simulink model "cal_2adc"  (R2012b)
settings: Solver=ode45  StartTime=0.0  StopTime=10.0  RelTol=1e-3
libraries: xbsIndex_r4 x665, dspsigops x32, xps_library x1
(part 1 of 5)
settings Model: Creator=rprimian  LastModifiedBy=root
settings DataIOCC: SignalLoggingSaveFormat=ModelDataLogs
settings DebuggingCC: SolverPrmCheckMsg=none  FcnCallInpInsideContextMsg=UseLocalSettings  StrictBusMsg=Warning
settings GRTTargetCC: CombineOutputUpdateFcns=off  GRTInterface=on

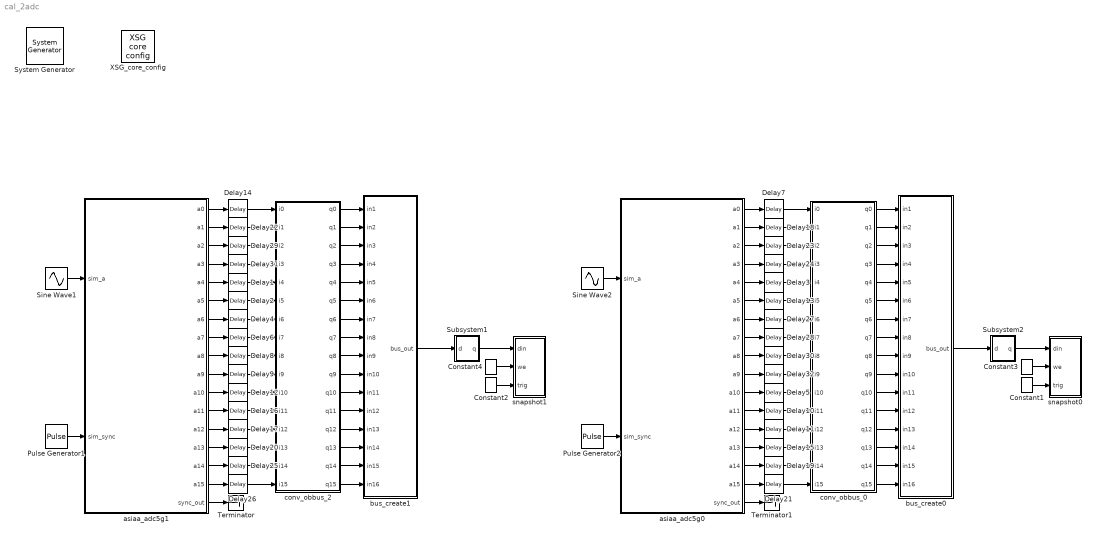
== system cal_2adc ==
  " System Generator" : xbsIndex_r4/ System Generator  Tag=genX  xilinxfamily=virtex6  part=xc6vsx475t  speed=-1  package=ff1759  synthesis_tool=XST  clock_wrapper=Clock Enables  directory=./cal_2adc/sysgen  proj_type=Project Navigator  Synth_file=XST Defaults  Impl_file=ISE Defaults  testbench=off  simulink_period=1  sysclk_period=4  dcm_input_clock_period=100  incr_netlist=off  trim_vbits=Everywhere in SubSystem  dbl_ovrd=According to Block Masks  core_generation=According to Block Masks  run_coregen=off  deprecated_control=off  eval_field=0  block_type=sysgen
  Constant{1..4} (4 alike) : xbsIndex_r4/Constant  const=1  gui_display_data_type=Fixed-point  arith_type=Boolean  n_bits=16  bin_pt=14  preci_type=Single  exp_width=8  frac_width=24  explicit_period=on  period=1  equ=P=C  opselect=C  inp2=PCIN>>17  opr=+  inp1=P  carry=CIN  dbl_ovrd=off  block_type=constant
      settings: block_version=11.4
  Delay{1..32} (32 alike) : xbsIndex_r4/Delay  rst=off  infoeditControl=Selection of Reset will increase slice count due to use of real FFs and instead of SRLs  en=off  latency=2  dbl_ovrd=off  reg_retiming=off  block_type=delay
  Pulse Generator1 : DiscretePulseGenerator  Period=1000
  Pulse Generator2 : DiscretePulseGenerator  Period=1000
  Sine Wave1 : Sin  SineType=Sample based  SampleTime=1/8
  Sine Wave2 : Sin  SineType=Sample based  SampleTime=1/8
  Subsystem1 : Subsystem
  Subsystem2 : Subsystem
  Terminator : Terminator
  Terminator1 : Terminator
  XSG_core_config : xps_library/XSG core config  Tag=xps:xsg  hw_sys=ROACH2:sx475t  clk_src=adc1_clk  ROACH_clk_src=adc0_clk  ROACH2_clk_src=adc1_clk  clk_rate=250  sample_period=1  synthesis_tool=XST
  asiaa_adc5g0 : Subsystem  Tag=xps:adc5g  AncestorBlock=xps_library/ADCs/asiaa_adc5g  mask(adc5g){input_mode=One-channel -- A, adc_brd=ZDOK 0, demux=1:1, adc_bit_width=8, adc_clk_rate=1200, using_ctrl=on, test_ramp=off}
      mask prompts: input_mode "Input mode:"; adc_brd "ADC Board"; demux "Internal demux"; adc_bit_width "ADC Resolution (bits):"; adc_clk_rate "ADC Clock Rate (MHz):"; using_ctrl "use control"; test_ramp "start in test ramp mode"
      mask help:
      | Interface for the ASIAA 5 GSps ADC. Supports interleaving all four
      | cores using either input A or C, or interleaving two-cores each for
      | A and C. The hardware itself comes in two versions:
      |
      | DMUX 1:2 -- 4-bit samples, 4 parallel streams
      | DMUX 1:1 -- 8-bit samples, 2 parallel streams
      |
      | In either configuration this block will output 8 parallel streams
      | but the underlying interface, and the bitwidth of the samples,
      | will be different.
      mask init:
      | adc5g_init(gcb,...
      |     'input_mode', input_mode,...
      |     'demux', demux,...
      |     'adc_clk_rate', adc_clk_rate,...
      |     'adc_bit_width', adc_bit_width,...
      |     'adc_brd', adc_brd,...
      |     'using_ctrl', using_ctrl,...
      |     'test_ramp', test_ramp);
      mask TypeOptions input_mode: One-channel -- A | One-channel -- C | Two-channel -- A&C
      mask TypeOptions adc_brd: ZDOK 0 | ZDOK 1
      mask TypeOptions demux: 1:1 | 1:2
      mask Callback demux:
      | demux = get_param(gcb,'demux');
      | if(strcmp(demux,'1:1')),
      |     set_param(gcb, 'adc_bit_width', '8')
      | elseif(strcmp(demux, '1:2')),
      |     set_param(gcb, 'adc_bit_width', '4');
      | else
      | end
  asiaa_adc5g1 : Subsystem  Tag=xps:adc5g  AncestorBlock=xps_library/ADCs/asiaa_adc5g  mask(adc5g){input_mode=One-channel -- A, adc_brd=ZDOK 1, demux=1:1, adc_bit_width=8, adc_clk_rate=1800, using_ctrl=on, test_ramp=off}
      mask prompts: input_mode "Input mode:"; adc_brd "ADC Board"; demux "Internal demux"; adc_bit_width "ADC Resolution (bits):"; adc_clk_rate "ADC Clock Rate (MHz):"; using_ctrl "use control"; test_ramp "start in test ramp mode"
      mask help:
      | Interface for the ASIAA 5 GSps ADC. Supports interleaving all four
      | cores using either input A or C, or interleaving two-cores each for
      | A and C. The hardware itself comes in two versions:
      |
      | DMUX 1:2 -- 4-bit samples, 4 parallel streams
      | DMUX 1:1 -- 8-bit samples, 2 parallel streams
      |
      | In either configuration this block will output 8 parallel streams
      | but the underlying interface, and the bitwidth of the samples,
      | will be different.
      mask init: same as cal_2adc/asiaa_adc5g0
      mask TypeOptions input_mode: One-channel -- A | One-channel -- C | Two-channel -- A&C
      mask TypeOptions adc_brd: ZDOK 0 | ZDOK 1
      mask TypeOptions demux: 1:1 | 1:2
      mask Callback demux:
      | demux = get_param(gcb,'demux');
      | if(strcmp(demux,'1:1')),
      |     set_param(gcb, 'adc_bit_width', '8')
      | elseif(strcmp(demux, '1:2')),
      |     set_param(gcb, 'adc_bit_width', '4');
      | else
      | end
  bus_create0 : Subsystem  AncestorBlock=casper_library_flow_control/bus_create  mask(bus_create){inputNum=16}
      mask prompts: inputNum "Number of inputs:"
      mask init:
      | bus_create_init(gcb,...
      |     'inputNum', inputNum);
  bus_create1 : Subsystem  AncestorBlock=casper_library_flow_control/bus_create  mask(bus_create){inputNum=16}
      mask prompts: inputNum "Number of inputs:"
      mask init:
      | bus_create_init(gcb,...
      |     'inputNum', inputNum);
  conv_obbus_0 : Subsystem
  conv_obbus_2 : Subsystem
  snapshot0 : Subsystem  Tag=casper:snapshot  AncestorBlock=casper_library_scopes/snapshot  mask(snapshot){storage=bram, dram_dimm=1, dram_clock=200, nsamples=10, data_width=128, offset=on, circap=off, value=off, use_dsp48=on}
      mask prompts: storage "Storage medium"; dram_dimm "DRAM dimm"; dram_clock "DRAM clock rate"; nsamples "Number of Samples (2^?)"; data_width "Data width"; offset "Start delay support"; circap "Circular capture support"; value "Extra value capture support"; use_dsp48 "Use DSP48s to implement counters"
      mask help:
      | Standard snap block, but with the following optional extras;
      |  1) Optionally delay the fabric trigger by a user-specified number of valids.
      |  2) Capture continuously after a trigger until a stop pulse is received. Data is captured into BRAM continuously, with old data being overwritten until a stop command is received. Then stop capturing when memory is filled. This enables you to get some data before and some data after the stop pulse. Use the 'tr_en_cnt' register to determine where you are in your vector. 'Addr' register's MSb now indicates 'busy capturing'.
      |  3) Optionally capture a value on an input port to a register at the same time as the first data sample.
      |  4) Implement counters using DSP48Es to save resources.
      mask init:
      | snapshot_init(gcb, ...
      |     'storage', storage, ...
      |     'dram_dimm', dram_dimm, ...
      |     'dram_clock', dram_clock, ...
      |     'nsamples', nsamples, ...
      |     'data_width', data_width, ...
      |     'offset', offset, ...
      |     'circap', circap, ...
      |     'value', value, ...
      |     'use_dsp48', use_dsp48);
      mask TypeOptions storage: bram | dram
      mask Callback storage: snapshot_callback();
      mask TypeOptions dram_dimm: 1 | 2 | 3 | 4
      mask TypeOptions dram_clock: 200 | 250 | 266 | 300 | 333
      mask TypeOptions data_width: 8 | 16 | 32 | 64 | 128
  snapshot1 : Subsystem  Tag=casper:snapshot  AncestorBlock=casper_library_scopes/snapshot  mask(snapshot){storage=bram, dram_dimm=1, dram_clock=200, nsamples=10, data_width=128, offset=on, circap=off, value=off, use_dsp48=on}
      mask prompts: storage "Storage medium"; dram_dimm "DRAM dimm"; dram_clock "DRAM clock rate"; nsamples "Number of Samples (2^?)"; data_width "Data width"; offset "Start delay support"; circap "Circular capture support"; value "Extra value capture support"; use_dsp48 "Use DSP48s to implement counters"
      mask help:
      | Standard snap block, but with the following optional extras;
      |  1) Optionally delay the fabric trigger by a user-specified number of valids.
      |  2) Capture continuously after a trigger until a stop pulse is received. Data is captured into BRAM continuously, with old data being overwritten until a stop command is received. Then stop capturing when memory is filled. This enables you to get some data before and some data after the stop pulse. Use the 'tr_en_cnt' register to determine where you are in your vector. 'Addr' register's MSb now indicates 'busy capturing'.
      |  3) Optionally capture a value on an input port to a register at the same time as the first data sample.
      |  4) Implement counters using DSP48Es to save resources.
      mask init: same as cal_2adc/snapshot0
      mask TypeOptions storage: bram | dram
      mask Callback storage: snapshot_callback();
      mask TypeOptions dram_dimm: 1 | 2 | 3 | 4
      mask TypeOptions dram_clock: 200 | 250 | 266 | 300 | 333
      mask TypeOptions data_width: 8 | 16 | 32 | 64 | 128
  wires:
  Constant4/1 -> snapshot1/2(we)
  Pulse Generator1/1 -> asiaa_adc5g1/2(sim_sync)
  Sine Wave1/1 -> asiaa_adc5g1/1(sim_a)
  Subsystem1/1(q) -> snapshot1/1(din)
  Constant2/1 -> snapshot1/3(trig)
  asiaa_adc5g1/17(sync_out) -> Terminator/1
  asiaa_adc5g1/11(a10) -> Delay12/1
  asiaa_adc5g1/12(a11) -> Delay16/1
  asiaa_adc5g1/13(a12) -> Delay17/1
  asiaa_adc5g1/14(a13) -> Delay20/1
  asiaa_adc5g1/1(a0) -> Delay14/1
  asiaa_adc5g1/2(a1) -> Delay22/1
  asiaa_adc5g1/3(a2) -> Delay29/1
  asiaa_adc5g1/4(a3) -> Delay31/1
  asiaa_adc5g1/5(a4) -> Delay1/1
  asiaa_adc5g1/6(a5) -> Delay2/1
  asiaa_adc5g1/7(a6) -> Delay4/1
  asiaa_adc5g1/8(a7) -> Delay6/1
  asiaa_adc5g1/9(a8) -> Delay8/1
  asiaa_adc5g1/10(a9) -> Delay9/1
  asiaa_adc5g1/15(a14) -> Delay25/1
  asiaa_adc5g1/16(a15) -> Delay26/1
  bus_create1/1(bus_out) -> Subsystem1/1(d)
  Delay29/1 -> conv_obbus_2/3(i2)
  Delay8/1 -> conv_obbus_2/9(i8)
  Delay4/1 -> conv_obbus_2/7(i6)
  Delay9/1 -> conv_obbus_2/10(i9)
  Delay6/1 -> conv_obbus_2/8(i7)
  Delay16/1 -> conv_obbus_2/12(i11)
  Delay12/1 -> conv_obbus_2/11(i10)
  Delay17/1 -> conv_obbus_2/13(i12)
  Delay2/1 -> conv_obbus_2/6(i5)
  Delay22/1 -> conv_obbus_2/2(i1)
  Delay20/1 -> conv_obbus_2/14(i13)
  Delay31/1 -> conv_obbus_2/4(i3)
  Delay14/1 -> conv_obbus_2/1(i0)
  Delay25/1 -> conv_obbus_2/15(i14)
  Delay26/1 -> conv_obbus_2/16(i15)
  Delay1/1 -> conv_obbus_2/5(i4)
  conv_obbus_2/5(q4) -> bus_create1/5(in5)
  conv_obbus_2/7(q6) -> bus_create1/7(in7)
  conv_obbus_2/2(q1) -> bus_create1/2(in2)
  conv_obbus_2/11(q10) -> bus_create1/11(in11)
  conv_obbus_2/8(q7) -> bus_create1/8(in8)
  conv_obbus_2/13(q12) -> bus_create1/13(in13)
  conv_obbus_2/4(q3) -> bus_create1/4(in4)
  conv_obbus_2/15(q14) -> bus_create1/15(in15)
  conv_obbus_2/16(q15) -> bus_create1/16(in16)
  conv_obbus_2/12(q11) -> bus_create1/12(in12)
  conv_obbus_2/6(q5) -> bus_create1/6(in6)
  conv_obbus_2/14(q13) -> bus_create1/14(in14)
  conv_obbus_2/1(q0) -> bus_create1/1(in1)
  conv_obbus_2/10(q9) -> bus_create1/10(in10)
  conv_obbus_2/9(q8) -> bus_create1/9(in9)
  conv_obbus_2/3(q2) -> bus_create1/3(in3)
  Constant3/1 -> snapshot0/2(we)
  Pulse Generator2/1 -> asiaa_adc5g0/2(sim_sync)
  Sine Wave2/1 -> asiaa_adc5g0/1(sim_a)
  Subsystem2/1(q) -> snapshot0/1(din)
  Constant1/1 -> snapshot0/3(trig)
  asiaa_adc5g0/17(sync_out) -> Terminator1/1
  asiaa_adc5g0/11(a10) -> Delay5/1
  asiaa_adc5g0/12(a11) -> Delay10/1
  asiaa_adc5g0/13(a12) -> Delay11/1
  asiaa_adc5g0/14(a13) -> Delay15/1
  asiaa_adc5g0/1(a0) -> Delay7/1
  asiaa_adc5g0/2(a1) -> Delay18/1
  asiaa_adc5g0/3(a2) -> Delay23/1
  asiaa_adc5g0/4(a3) -> Delay24/1
  asiaa_adc5g0/5(a4) -> Delay3/1
  asiaa_adc5g0/6(a5) -> Delay13/1
  asiaa_adc5g0/7(a6) -> Delay27/1
  asiaa_adc5g0/8(a7) -> Delay28/1
  asiaa_adc5g0/9(a8) -> Delay30/1
  asiaa_adc5g0/10(a9) -> Delay32/1
  asiaa_adc5g0/15(a14) -> Delay19/1
  asiaa_adc5g0/16(a15) -> Delay21/1
  bus_create0/1(bus_out) -> Subsystem2/1(d)
  Delay23/1 -> conv_obbus_0/3(i2)
  Delay30/1 -> conv_obbus_0/9(i8)
  Delay27/1 -> conv_obbus_0/7(i6)
  Delay32/1 -> conv_obbus_0/10(i9)
  Delay28/1 -> conv_obbus_0/8(i7)
  Delay10/1 -> conv_obbus_0/12(i11)
  Delay5/1 -> conv_obbus_0/11(i10)
  Delay11/1 -> conv_obbus_0/13(i12)
  Delay13/1 -> conv_obbus_0/6(i5)
  Delay18/1 -> conv_obbus_0/2(i1)
  Delay15/1 -> conv_obbus_0/14(i13)
  Delay24/1 -> conv_obbus_0/4(i3)
  Delay7/1 -> conv_obbus_0/1(i0)
  Delay19/1 -> conv_obbus_0/15(i14)
  Delay21/1 -> conv_obbus_0/16(i15)
  Delay3/1 -> conv_obbus_0/5(i4)
  conv_obbus_0/5(q4) -> bus_create0/5(in5)
  conv_obbus_0/7(q6) -> bus_create0/7(in7)
  conv_obbus_0/2(q1) -> bus_create0/2(in2)
  conv_obbus_0/11(q10) -> bus_create0/11(in11)
  conv_obbus_0/8(q7) -> bus_create0/8(in8)
  conv_obbus_0/13(q12) -> bus_create0/13(in13)
  conv_obbus_0/4(q3) -> bus_create0/4(in4)
  conv_obbus_0/15(q14) -> bus_create0/15(in15)
  conv_obbus_0/16(q15) -> bus_create0/16(in16)
  conv_obbus_0/12(q11) -> bus_create0/12(in12)
  conv_obbus_0/6(q5) -> bus_create0/6(in6)
  conv_obbus_0/14(q13) -> bus_create0/14(in14)
  conv_obbus_0/1(q0) -> bus_create0/1(in1)
  conv_obbus_0/10(q9) -> bus_create0/10(in10)
  conv_obbus_0/9(q8) -> bus_create0/9(in9)
  conv_obbus_0/3(q2) -> bus_create0/3(in3)

== system cal_2adc/Subsystem1 ==
  d : Inport
  Register : xbsIndex_r4/Register  init=0  rst=off  en=off  dbl_ovrd=off  block_type=register
      settings: block_version=11.4
  Register1 : xbsIndex_r4/Register  init=0  rst=off  en=off  dbl_ovrd=off  block_type=register
      settings: block_version=11.4
  q : Outport
  wires:
  Register1/1 -> q/1
  Register/1 -> Register1/1
  d/1 -> Register/1

== system cal_2adc/Subsystem2 ==
  d : Inport
  Register : xbsIndex_r4/Register  init=0  rst=off  en=off  dbl_ovrd=off  block_type=register
      settings: block_version=11.4
  Register1 : xbsIndex_r4/Register  init=0  rst=off  en=off  dbl_ovrd=off  block_type=register
      settings: block_version=11.4
  q : Outport
  wires:
  d/1 -> Register/1
  Register/1 -> Register1/1
  Register1/1 -> q/1

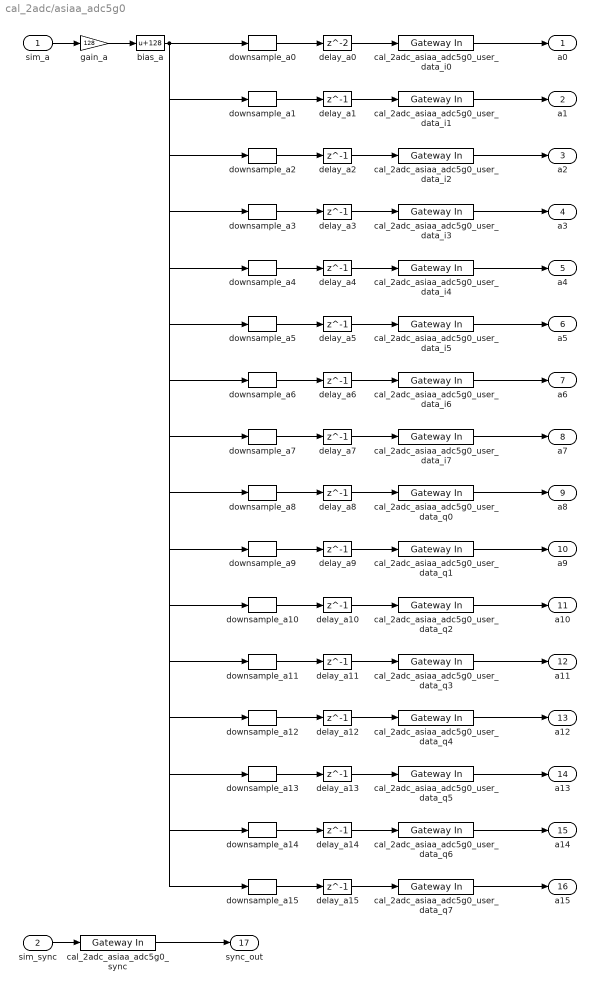
== system cal_2adc/asiaa_adc5g0 ==
  sim_a : Inport
  sim_sync : Inport  Port=2
  bias_a : Bias  Bias=128  SaturateOnIntegerOverflow=on
  cal_2adc_asiaa_adc5g0_sync : xbsIndex_r4/Gateway In  gui_display_data_type=Fixed-point  arith_type=Boolean  n_bits=16  bin_pt=14  preci_type=Single  exp_width=8  frac_width=24  quantization="Round  (unbiased: +/- Inf)"  overflow=Saturate  period=1  dbl_ovrd=off  timing_constraint=None  locs_specified=off  LOCs={}  UseAsADC=off  ADCChannel='1'  inherit_from_input=off  hdl_port=on  block_type=gatewayin
  cal_2adc_asiaa_adc5g0_user_data_i{0..7} (8 alike) : xbsIndex_r4/Gateway In  gui_display_data_type=Fixed-point  arith_type=Unsigned  n_bits=8  bin_pt=0  preci_type=Single  exp_width=8  frac_width=24  quantization=Truncate  overflow=Wrap  period=1  dbl_ovrd=off  timing_constraint=None  locs_specified=off  LOCs={}  UseAsADC=off  ADCChannel='1'  inherit_from_input=off  hdl_port=on  block_type=gatewayin
  cal_2adc_asiaa_adc5g0_user_data_q{0..7} (8 alike) : xbsIndex_r4/Gateway In  gui_display_data_type=Fixed-point  arith_type=Unsigned  n_bits=8  bin_pt=0  preci_type=Single  exp_width=8  frac_width=24  quantization=Truncate  overflow=Wrap  period=1  dbl_ovrd=off  timing_constraint=None  locs_specified=off  LOCs={}  UseAsADC=off  ADCChannel='1'  inherit_from_input=off  hdl_port=on  block_type=gatewayin
  delay_a0 : Delay  InitialCondition=0  InputProcessing=Inherited
  delay_a{1..15} (15 alike) : Delay  DelayLength=1  InitialCondition=0  InputProcessing=Inherited
  downsample_a0 : dspsigops/Downsample  N=16  phase=0  RateOptions=Allow multirate processing  smode=Allow multirate  fmode=Maintain input frame size  ic=0
  downsample_a1 : dspsigops/Downsample  N=16  phase=1  RateOptions=Allow multirate processing  smode=Allow multirate  fmode=Maintain input frame size  ic=0
  downsample_a10 : dspsigops/Downsample  N=16  phase=10  RateOptions=Allow multirate processing  smode=Allow multirate  fmode=Maintain input frame size  ic=0
  downsample_a11 : dspsigops/Downsample  N=16  phase=11  RateOptions=Allow multirate processing  smode=Allow multirate  fmode=Maintain input frame size  ic=0
  downsample_a12 : dspsigops/Downsample  N=16  phase=12  RateOptions=Allow multirate processing  smode=Allow multirate  fmode=Maintain input frame size  ic=0
  downsample_a13 : dspsigops/Downsample  N=16  phase=13  RateOptions=Allow multirate processing  smode=Allow multirate  fmode=Maintain input frame size  ic=0
  downsample_a14 : dspsigops/Downsample  N=16  phase=14  RateOptions=Allow multirate processing  smode=Allow multirate  fmode=Maintain input frame size  ic=0
  downsample_a15 : dspsigops/Downsample  N=16  phase=15  RateOptions=Allow multirate processing  smode=Allow multirate  fmode=Maintain input frame size  ic=0
  downsample_a2 : dspsigops/Downsample  N=16  phase=2  RateOptions=Allow multirate processing  smode=Allow multirate  fmode=Maintain input frame size  ic=0
  downsample_a3 : dspsigops/Downsample  N=16  phase=3  RateOptions=Allow multirate processing  smode=Allow multirate  fmode=Maintain input frame size  ic=0
  downsample_a4 : dspsigops/Downsample  N=16  phase=4  RateOptions=Allow multirate processing  smode=Allow multirate  fmode=Maintain input frame size  ic=0
  downsample_a5 : dspsigops/Downsample  N=16  phase=5  RateOptions=Allow multirate processing  smode=Allow multirate  fmode=Maintain input frame size  ic=0
  downsample_a6 : dspsigops/Downsample  N=16  phase=6  RateOptions=Allow multirate processing  smode=Allow multirate  fmode=Maintain input frame size  ic=0
  downsample_a7 : dspsigops/Downsample  N=16  phase=7  RateOptions=Allow multirate processing  smode=Allow multirate  fmode=Maintain input frame size  ic=0
  downsample_a8 : dspsigops/Downsample  N=16  phase=8  RateOptions=Allow multirate processing  smode=Allow multirate  fmode=Maintain input frame size  ic=0
  downsample_a9 : dspsigops/Downsample  N=16  phase=9  RateOptions=Allow multirate processing  smode=Allow multirate  fmode=Maintain input frame size  ic=0
  gain_a : Gain  Gain=128  SaturateOnIntegerOverflow=on  OutDataTypeStr=Inherit: Same as input  ParamDataTypeStr=Inherit: Same as input
  a0 : Outport
  a1 : Outport  Port=2
  a2 : Outport  Port=3
  a3 : Outport  Port=4
  a4 : Outport  Port=5
  a5 : Outport  Port=6
  a6 : Outport  Port=7
  a7 : Outport  Port=8
  a8 : Outport  Port=9
  a9 : Outport  Port=10
  a10 : Outport  Port=11
  a11 : Outport  Port=12
  a12 : Outport  Port=13
  a13 : Outport  Port=14
  a14 : Outport  Port=15
  a15 : Outport  Port=16
  sync_out : Outport  Port=17
  wires:
  sim_a/1 -> gain_a/1
  gain_a/1 -> bias_a/1
  bias_a/1 -> downsample_a0/1, downsample_a1/1, downsample_a2/1, downsample_a3/1, downsample_a4/1, downsample_a5/1, downsample_a6/1, downsample_a7/1, downsample_a8/1, downsample_a9/1, downsample_a10/1, downsample_a11/1, downsample_a12/1, downsample_a13/1, downsample_a14/1, downsample_a15/1
  downsample_a0/1 -> delay_a0/1
  delay_a0/1 -> cal_2adc_asiaa_adc5g0_user_data_i0/1
  cal_2adc_asiaa_adc5g0_user_data_i0/1 -> a0/1
  downsample_a1/1 -> delay_a1/1
  delay_a1/1 -> cal_2adc_asiaa_adc5g0_user_data_i1/1
  cal_2adc_asiaa_adc5g0_user_data_i1/1 -> a1/1
  downsample_a2/1 -> delay_a2/1
  delay_a2/1 -> cal_2adc_asiaa_adc5g0_user_data_i2/1
  cal_2adc_asiaa_adc5g0_user_data_i2/1 -> a2/1
  downsample_a3/1 -> delay_a3/1
  delay_a3/1 -> cal_2adc_asiaa_adc5g0_user_data_i3/1
  cal_2adc_asiaa_adc5g0_user_data_i3/1 -> a3/1
  downsample_a4/1 -> delay_a4/1
  delay_a4/1 -> cal_2adc_asiaa_adc5g0_user_data_i4/1
  cal_2adc_asiaa_adc5g0_user_data_i4/1 -> a4/1
  downsample_a5/1 -> delay_a5/1
  delay_a5/1 -> cal_2adc_asiaa_adc5g0_user_data_i5/1
  cal_2adc_asiaa_adc5g0_user_data_i5/1 -> a5/1
  downsample_a6/1 -> delay_a6/1
  delay_a6/1 -> cal_2adc_asiaa_adc5g0_user_data_i6/1
  cal_2adc_asiaa_adc5g0_user_data_i6/1 -> a6/1
  downsample_a7/1 -> delay_a7/1
  delay_a7/1 -> cal_2adc_asiaa_adc5g0_user_data_i7/1
  cal_2adc_asiaa_adc5g0_user_data_i7/1 -> a7/1
  downsample_a8/1 -> delay_a8/1
  delay_a8/1 -> cal_2adc_asiaa_adc5g0_user_data_q0/1
  cal_2adc_asiaa_adc5g0_user_data_q0/1 -> a8/1
  downsample_a9/1 -> delay_a9/1
  delay_a9/1 -> cal_2adc_asiaa_adc5g0_user_data_q1/1
  cal_2adc_asiaa_adc5g0_user_data_q1/1 -> a9/1
  downsample_a10/1 -> delay_a10/1
  delay_a10/1 -> cal_2adc_asiaa_adc5g0_user_data_q2/1
  cal_2adc_asiaa_adc5g0_user_data_q2/1 -> a10/1
  downsample_a11/1 -> delay_a11/1
  delay_a11/1 -> cal_2adc_asiaa_adc5g0_user_data_q3/1
  cal_2adc_asiaa_adc5g0_user_data_q3/1 -> a11/1
  downsample_a12/1 -> delay_a12/1
  delay_a12/1 -> cal_2adc_asiaa_adc5g0_user_data_q4/1
  cal_2adc_asiaa_adc5g0_user_data_q4/1 -> a12/1
  downsample_a13/1 -> delay_a13/1
  delay_a13/1 -> cal_2adc_asiaa_adc5g0_user_data_q5/1
  cal_2adc_asiaa_adc5g0_user_data_q5/1 -> a13/1
  downsample_a14/1 -> delay_a14/1
  delay_a14/1 -> cal_2adc_asiaa_adc5g0_user_data_q6/1
  cal_2adc_asiaa_adc5g0_user_data_q6/1 -> a14/1
  downsample_a15/1 -> delay_a15/1
  delay_a15/1 -> cal_2adc_asiaa_adc5g0_user_data_q7/1
  cal_2adc_asiaa_adc5g0_user_data_q7/1 -> a15/1
  sim_sync/1 -> cal_2adc_asiaa_adc5g0_sync/1
  cal_2adc_asiaa_adc5g0_sync/1 -> sync_out/1

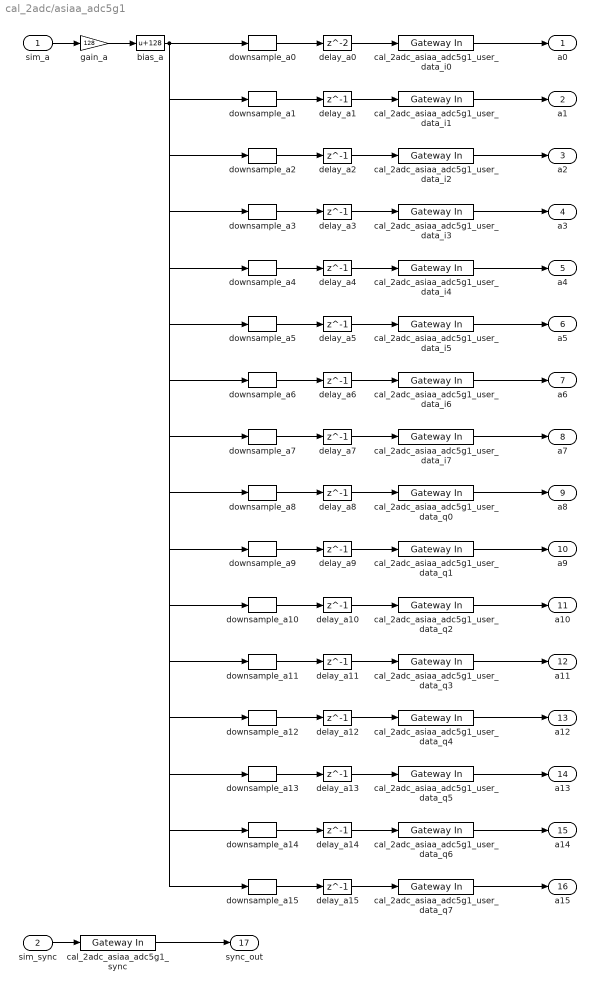
== system cal_2adc/asiaa_adc5g1 ==
  sim_a : Inport
  sim_sync : Inport  Port=2
  bias_a : Bias  Bias=128  SaturateOnIntegerOverflow=on
  cal_2adc_asiaa_adc5g1_sync : xbsIndex_r4/Gateway In  gui_display_data_type=Fixed-point  arith_type=Boolean  n_bits=16  bin_pt=14  preci_type=Single  exp_width=8  frac_width=24  quantization="Round  (unbiased: +/- Inf)"  overflow=Saturate  period=1  dbl_ovrd=off  timing_constraint=None  locs_specified=off  LOCs={}  UseAsADC=off  ADCChannel='1'  inherit_from_input=off  hdl_port=on  block_type=gatewayin
  cal_2adc_asiaa_adc5g1_user_data_i{0..7} (8 alike) : xbsIndex_r4/Gateway In  gui_display_data_type=Fixed-point  arith_type=Unsigned  n_bits=8  bin_pt=0  preci_type=Single  exp_width=8  frac_width=24  quantization=Truncate  overflow=Wrap  period=1  dbl_ovrd=off  timing_constraint=None  locs_specified=off  LOCs={}  UseAsADC=off  ADCChannel='1'  inherit_from_input=off  hdl_port=on  block_type=gatewayin
  cal_2adc_asiaa_adc5g1_user_data_q{0..7} (8 alike) : xbsIndex_r4/Gateway In  gui_display_data_type=Fixed-point  arith_type=Unsigned  n_bits=8  bin_pt=0  preci_type=Single  exp_width=8  frac_width=24  quantization=Truncate  overflow=Wrap  period=1  dbl_ovrd=off  timing_constraint=None  locs_specified=off  LOCs={}  UseAsADC=off  ADCChannel='1'  inherit_from_input=off  hdl_port=on  block_type=gatewayin
  delay_a0 : Delay  InitialCondition=0  InputProcessing=Inherited
  delay_a{1..15} (15 alike) : Delay  DelayLength=1  InitialCondition=0  InputProcessing=Inherited
  downsample_a0 : dspsigops/Downsample  N=16  phase=0  RateOptions=Allow multirate processing  smode=Allow multirate  fmode=Maintain input frame size  ic=0
  downsample_a1 : dspsigops/Downsample  N=16  phase=1  RateOptions=Allow multirate processing  smode=Allow multirate  fmode=Maintain input frame size  ic=0
  downsample_a10 : dspsigops/Downsample  N=16  phase=10  RateOptions=Allow multirate processing  smode=Allow multirate  fmode=Maintain input frame size  ic=0
  downsample_a11 : dspsigops/Downsample  N=16  phase=11  RateOptions=Allow multirate processing  smode=Allow multirate  fmode=Maintain input frame size  ic=0
  downsample_a12 : dspsigops/Downsample  N=16  phase=12  RateOptions=Allow multirate processing  smode=Allow multirate  fmode=Maintain input frame size  ic=0
  downsample_a13 : dspsigops/Downsample  N=16  phase=13  RateOptions=Allow multirate processing  smode=Allow multirate  fmode=Maintain input frame size  ic=0
  downsample_a14 : dspsigops/Downsample  N=16  phase=14  RateOptions=Allow multirate processing  smode=Allow multirate  fmode=Maintain input frame size  ic=0
  downsample_a15 : dspsigops/Downsample  N=16  phase=15  RateOptions=Allow multirate processing  smode=Allow multirate  fmode=Maintain input frame size  ic=0
  downsample_a2 : dspsigops/Downsample  N=16  phase=2  RateOptions=Allow multirate processing  smode=Allow multirate  fmode=Maintain input frame size  ic=0
  downsample_a3 : dspsigops/Downsample  N=16  phase=3  RateOptions=Allow multirate processing  smode=Allow multirate  fmode=Maintain input frame size  ic=0
  downsample_a4 : dspsigops/Downsample  N=16  phase=4  RateOptions=Allow multirate processing  smode=Allow multirate  fmode=Maintain input frame size  ic=0
  downsample_a5 : dspsigops/Downsample  N=16  phase=5  RateOptions=Allow multirate processing  smode=Allow multirate  fmode=Maintain input frame size  ic=0
  downsample_a6 : dspsigops/Downsample  N=16  phase=6  RateOptions=Allow multirate processing  smode=Allow multirate  fmode=Maintain input frame size  ic=0
  downsample_a7 : dspsigops/Downsample  N=16  phase=7  RateOptions=Allow multirate processing  smode=Allow multirate  fmode=Maintain input frame size  ic=0
  downsample_a8 : dspsigops/Downsample  N=16  phase=8  RateOptions=Allow multirate processing  smode=Allow multirate  fmode=Maintain input frame size  ic=0
  downsample_a9 : dspsigops/Downsample  N=16  phase=9  RateOptions=Allow multirate processing  smode=Allow multirate  fmode=Maintain input frame size  ic=0
  gain_a : Gain  Gain=128  SaturateOnIntegerOverflow=on  OutDataTypeStr=Inherit: Same as input  ParamDataTypeStr=Inherit: Same as input
  a0 : Outport
  a1 : Outport  Port=2
  a2 : Outport  Port=3
  a3 : Outport  Port=4
  a4 : Outport  Port=5
  a5 : Outport  Port=6
  a6 : Outport  Port=7
  a7 : Outport  Port=8
  a8 : Outport  Port=9
  a9 : Outport  Port=10
  a10 : Outport  Port=11
  a11 : Outport  Port=12
  a12 : Outport  Port=13
  a13 : Outport  Port=14
  a14 : Outport  Port=15
  a15 : Outport  Port=16
  sync_out : Outport  Port=17
  wires:
  sim_a/1 -> gain_a/1
  gain_a/1 -> bias_a/1
  bias_a/1 -> downsample_a0/1, downsample_a1/1, downsample_a2/1, downsample_a3/1, downsample_a4/1, downsample_a5/1, downsample_a6/1, downsample_a7/1, downsample_a8/1, downsample_a9/1, downsample_a10/1, downsample_a11/1, downsample_a12/1, downsample_a13/1, downsample_a14/1, downsample_a15/1
  downsample_a0/1 -> delay_a0/1
  delay_a0/1 -> cal_2adc_asiaa_adc5g1_user_data_i0/1
  cal_2adc_asiaa_adc5g1_user_data_i0/1 -> a0/1
  downsample_a1/1 -> delay_a1/1
  delay_a1/1 -> cal_2adc_asiaa_adc5g1_user_data_i1/1
  cal_2adc_asiaa_adc5g1_user_data_i1/1 -> a1/1
  downsample_a2/1 -> delay_a2/1
  delay_a2/1 -> cal_2adc_asiaa_adc5g1_user_data_i2/1
  cal_2adc_asiaa_adc5g1_user_data_i2/1 -> a2/1
  downsample_a3/1 -> delay_a3/1
  delay_a3/1 -> cal_2adc_asiaa_adc5g1_user_data_i3/1
  cal_2adc_asiaa_adc5g1_user_data_i3/1 -> a3/1
  downsample_a4/1 -> delay_a4/1
  delay_a4/1 -> cal_2adc_asiaa_adc5g1_user_data_i4/1
  cal_2adc_asiaa_adc5g1_user_data_i4/1 -> a4/1
  downsample_a5/1 -> delay_a5/1
  delay_a5/1 -> cal_2adc_asiaa_adc5g1_user_data_i5/1
  cal_2adc_asiaa_adc5g1_user_data_i5/1 -> a5/1
  downsample_a6/1 -> delay_a6/1
  delay_a6/1 -> cal_2adc_asiaa_adc5g1_user_data_i6/1
  cal_2adc_asiaa_adc5g1_user_data_i6/1 -> a6/1
  downsample_a7/1 -> delay_a7/1
  delay_a7/1 -> cal_2adc_asiaa_adc5g1_user_data_i7/1
  cal_2adc_asiaa_adc5g1_user_data_i7/1 -> a7/1
  downsample_a8/1 -> delay_a8/1
  delay_a8/1 -> cal_2adc_asiaa_adc5g1_user_data_q0/1
  cal_2adc_asiaa_adc5g1_user_data_q0/1 -> a8/1
  downsample_a9/1 -> delay_a9/1
  delay_a9/1 -> cal_2adc_asiaa_adc5g1_user_data_q1/1
  cal_2adc_asiaa_adc5g1_user_data_q1/1 -> a9/1
  downsample_a10/1 -> delay_a10/1
  delay_a10/1 -> cal_2adc_asiaa_adc5g1_user_data_q2/1
  cal_2adc_asiaa_adc5g1_user_data_q2/1 -> a10/1
  downsample_a11/1 -> delay_a11/1
  delay_a11/1 -> cal_2adc_asiaa_adc5g1_user_data_q3/1
  cal_2adc_asiaa_adc5g1_user_data_q3/1 -> a11/1
  downsample_a12/1 -> delay_a12/1
  delay_a12/1 -> cal_2adc_asiaa_adc5g1_user_data_q4/1
  cal_2adc_asiaa_adc5g1_user_data_q4/1 -> a12/1
  downsample_a13/1 -> delay_a13/1
  delay_a13/1 -> cal_2adc_asiaa_adc5g1_user_data_q5/1
  cal_2adc_asiaa_adc5g1_user_data_q5/1 -> a13/1
  downsample_a14/1 -> delay_a14/1
  delay_a14/1 -> cal_2adc_asiaa_adc5g1_user_data_q6/1
  cal_2adc_asiaa_adc5g1_user_data_q6/1 -> a14/1
  downsample_a15/1 -> delay_a15/1
  delay_a15/1 -> cal_2adc_asiaa_adc5g1_user_data_q7/1
  cal_2adc_asiaa_adc5g1_user_data_q7/1 -> a15/1
  sim_sync/1 -> cal_2adc_asiaa_adc5g1_sync/1
  cal_2adc_asiaa_adc5g1_sync/1 -> sync_out/1

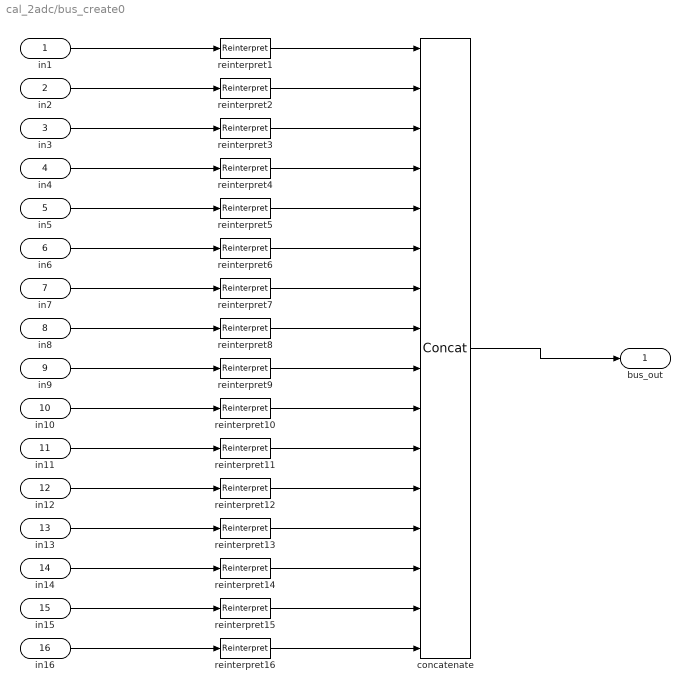
== system cal_2adc/bus_create0 ==
  in1 : Inport
  in2 : Inport  Port=2
  in3 : Inport  Port=3
  in4 : Inport  Port=4
  in5 : Inport  Port=5
  in6 : Inport  Port=6
  in7 : Inport  Port=7
  in8 : Inport  Port=8
  in9 : Inport  Port=9
  in10 : Inport  Port=10
  in11 : Inport  Port=11
  in12 : Inport  Port=12
  in13 : Inport  Port=13
  in14 : Inport  Port=14
  in15 : Inport  Port=15
  in16 : Inport  Port=16
  concatenate : xbsIndex_r4/Concat  num_inputs=16  dbl_ovrd=off  block_type=concat
  reinterpret{1..16} (16 alike) : xbsIndex_r4/Reinterpret  force_arith_type=on  arith_type=Unsigned  force_bin_pt=on  bin_pt=0  block_type=reinterpret
      reinterpret1 settings: infoedit="Changes signal type without altering the binary representation.   You can changed the signal between signed and unsigned, and relocate the binary point.<br><br>Hardware notes: In hardware this block costs nothing.<br><br>Example:  Suppose the input is 6 bits wide, signed, with 2 fractional bits, and the output is forced to unsigned with 0 fractional bits.  Then an input of -2.0 (1110.00 in binary 2's complement) becomes an output of 56 (111000 in binary)."
      reinterpret2 settings: infoedit="Changes signal type without altering the binary representation.   You can changed the signal between signed and unsigned, and relocate the binary point.<br><br>Hardware notes: In hardware this block costs nothing.<br><br>Example:  Suppose the input is 6 bits wide, signed, with 2 fractional bits, and the output is forced to unsigned with 0 fractional bits.  Then an input of -2.0 (1110.00 in binary 2's complement) becomes an output of 56 (111000 in binary)."
  bus_out : Outport
  wires:
  reinterpret16/1 -> concatenate/16
  in16/1 -> reinterpret16/1
  reinterpret15/1 -> concatenate/15
  in15/1 -> reinterpret15/1
  reinterpret14/1 -> concatenate/14
  in14/1 -> reinterpret14/1
  reinterpret13/1 -> concatenate/13
  in13/1 -> reinterpret13/1
  reinterpret12/1 -> concatenate/12
  in12/1 -> reinterpret12/1
  reinterpret11/1 -> concatenate/11
  in11/1 -> reinterpret11/1
  reinterpret10/1 -> concatenate/10
  in10/1 -> reinterpret10/1
  reinterpret9/1 -> concatenate/9
  in9/1 -> reinterpret9/1
  reinterpret8/1 -> concatenate/8
  in8/1 -> reinterpret8/1
  reinterpret7/1 -> concatenate/7
  in7/1 -> reinterpret7/1
  reinterpret6/1 -> concatenate/6
  in6/1 -> reinterpret6/1
  reinterpret5/1 -> concatenate/5
  in5/1 -> reinterpret5/1
  reinterpret4/1 -> concatenate/4
  in4/1 -> reinterpret4/1
  reinterpret3/1 -> concatenate/3
  in3/1 -> reinterpret3/1
  reinterpret2/1 -> concatenate/2
  in2/1 -> reinterpret2/1
  reinterpret1/1 -> concatenate/1
  in1/1 -> reinterpret1/1
  concatenate/1 -> bus_out/1

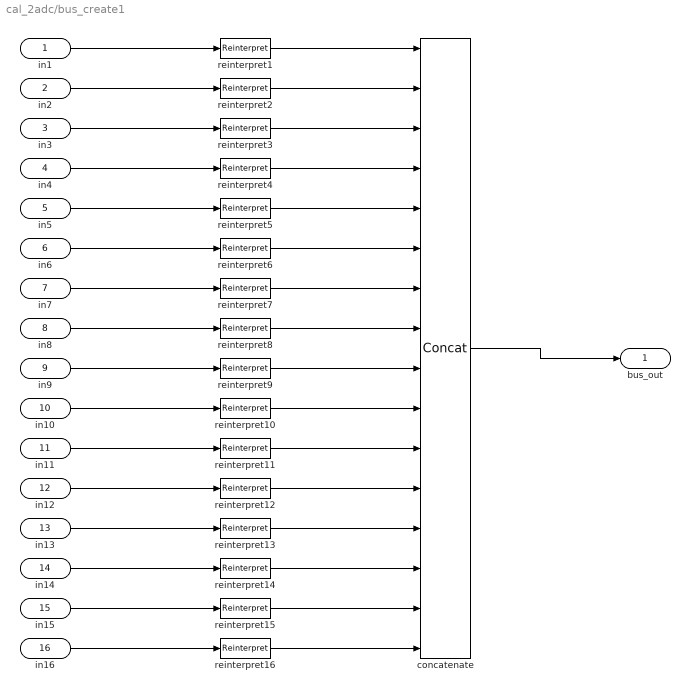
== system cal_2adc/bus_create1 ==
  in1 : Inport
  in2 : Inport  Port=2
  in3 : Inport  Port=3
  in4 : Inport  Port=4
  in5 : Inport  Port=5
  in6 : Inport  Port=6
  in7 : Inport  Port=7
  in8 : Inport  Port=8
  in9 : Inport  Port=9
  in10 : Inport  Port=10
  in11 : Inport  Port=11
  in12 : Inport  Port=12
  in13 : Inport  Port=13
  in14 : Inport  Port=14
  in15 : Inport  Port=15
  in16 : Inport  Port=16
  concatenate : xbsIndex_r4/Concat  num_inputs=16  dbl_ovrd=off  block_type=concat
  reinterpret{1..16} (16 alike) : xbsIndex_r4/Reinterpret  force_arith_type=on  arith_type=Unsigned  force_bin_pt=on  bin_pt=0  block_type=reinterpret
      reinterpret1 settings: infoedit="Changes signal type without altering the binary representation.   You can changed the signal between signed and unsigned, and relocate the binary point.<br><br>Hardware notes: In hardware this block costs nothing.<br><br>Example:  Suppose the input is 6 bits wide, signed, with 2 fractional bits, and the output is forced to unsigned with 0 fractional bits.  Then an input of -2.0 (1110.00 in binary 2's complement) becomes an output of 56 (111000 in binary)."
      reinterpret2 settings: infoedit="Changes signal type without altering the binary representation.   You can changed the signal between signed and unsigned, and relocate the binary point.<br><br>Hardware notes: In hardware this block costs nothing.<br><br>Example:  Suppose the input is 6 bits wide, signed, with 2 fractional bits, and the output is forced to unsigned with 0 fractional bits.  Then an input of -2.0 (1110.00 in binary 2's complement) becomes an output of 56 (111000 in binary)."
  bus_out : Outport
  wires:
  concatenate/1 -> bus_out/1
  in1/1 -> reinterpret1/1
  reinterpret1/1 -> concatenate/1
  in2/1 -> reinterpret2/1
  reinterpret2/1 -> concatenate/2
  in3/1 -> reinterpret3/1
  reinterpret3/1 -> concatenate/3
  in4/1 -> reinterpret4/1
  reinterpret4/1 -> concatenate/4
  in5/1 -> reinterpret5/1
  reinterpret5/1 -> concatenate/5
  in6/1 -> reinterpret6/1
  reinterpret6/1 -> concatenate/6
  in7/1 -> reinterpret7/1
  reinterpret7/1 -> concatenate/7
  in8/1 -> reinterpret8/1
  reinterpret8/1 -> concatenate/8
  in9/1 -> reinterpret9/1
  reinterpret9/1 -> concatenate/9
  in10/1 -> reinterpret10/1
  reinterpret10/1 -> concatenate/10
  in11/1 -> reinterpret11/1
  reinterpret11/1 -> concatenate/11
  in12/1 -> reinterpret12/1
  reinterpret12/1 -> concatenate/12
  in13/1 -> reinterpret13/1
  reinterpret13/1 -> concatenate/13
  in14/1 -> reinterpret14/1
  reinterpret14/1 -> concatenate/14
  in15/1 -> reinterpret15/1
  reinterpret15/1 -> concatenate/15
  in16/1 -> reinterpret16/1
  reinterpret16/1 -> concatenate/16

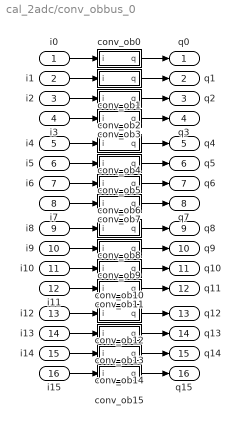
== system cal_2adc/conv_obbus_0 ==
  i0 : Inport
  i1 : Inport  Port=2
  i2 : Inport  Port=3
  i3 : Inport  Port=4
  i4 : Inport  Port=5
  i5 : Inport  Port=6
  i6 : Inport  Port=7
  i7 : Inport  Port=8
  i8 : Inport  Port=9
  i9 : Inport  Port=10
  i10 : Inport  Port=11
  i11 : Inport  Port=12
  i12 : Inport  Port=13
  i13 : Inport  Port=14
  i14 : Inport  Port=15
  i15 : Inport  Port=16
  conv_ob0 : Subsystem
  conv_ob1 : Subsystem
  conv_ob10 : Subsystem
  conv_ob11 : Subsystem
  conv_ob12 : Subsystem
  conv_ob13 : Subsystem
  conv_ob14 : Subsystem
  conv_ob15 : Subsystem
  conv_ob2 : Subsystem
  conv_ob3 : Subsystem
  conv_ob4 : Subsystem
  conv_ob5 : Subsystem
  conv_ob6 : Subsystem
  conv_ob7 : Subsystem
  conv_ob8 : Subsystem
  conv_ob9 : Subsystem
  q0 : Outport
  q1 : Outport  Port=2
  q2 : Outport  Port=3
  q3 : Outport  Port=4
  q4 : Outport  Port=5
  q5 : Outport  Port=6
  q6 : Outport  Port=7
  q7 : Outport  Port=8
  q8 : Outport  Port=9
  q9 : Outport  Port=10
  q10 : Outport  Port=11
  q11 : Outport  Port=12
  q12 : Outport  Port=13
  q13 : Outport  Port=14
  q14 : Outport  Port=15
  q15 : Outport  Port=16
  wires:
  conv_ob15/1(q) -> q15/1
  i15/1 -> conv_ob15/1(i)
  conv_ob14/1(q) -> q14/1
  i14/1 -> conv_ob14/1(i)
  conv_ob13/1(q) -> q13/1
  i13/1 -> conv_ob13/1(i)
  conv_ob12/1(q) -> q12/1
  i12/1 -> conv_ob12/1(i)
  conv_ob11/1(q) -> q11/1
  i11/1 -> conv_ob11/1(i)
  conv_ob10/1(q) -> q10/1
  i10/1 -> conv_ob10/1(i)
  conv_ob9/1(q) -> q9/1
  i9/1 -> conv_ob9/1(i)
  conv_ob8/1(q) -> q8/1
  i8/1 -> conv_ob8/1(i)
  conv_ob7/1(q) -> q7/1
  i7/1 -> conv_ob7/1(i)
  conv_ob6/1(q) -> q6/1
  i6/1 -> conv_ob6/1(i)
  conv_ob5/1(q) -> q5/1
  i5/1 -> conv_ob5/1(i)
  conv_ob4/1(q) -> q4/1
  i4/1 -> conv_ob4/1(i)
  conv_ob3/1(q) -> q3/1
  i3/1 -> conv_ob3/1(i)
  conv_ob2/1(q) -> q2/1
  i2/1 -> conv_ob2/1(i)
  conv_ob1/1(q) -> q1/1
  i1/1 -> conv_ob1/1(i)
  conv_ob0/1(q) -> q0/1
  i0/1 -> conv_ob0/1(i)

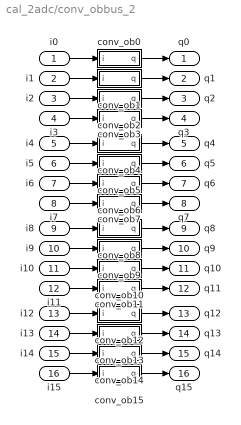
== system cal_2adc/conv_obbus_2 ==
  i0 : Inport
  i1 : Inport  Port=2
  i2 : Inport  Port=3
  i3 : Inport  Port=4
  i4 : Inport  Port=5
  i5 : Inport  Port=6
  i6 : Inport  Port=7
  i7 : Inport  Port=8
  i8 : Inport  Port=9
  i9 : Inport  Port=10
  i10 : Inport  Port=11
  i11 : Inport  Port=12
  i12 : Inport  Port=13
  i13 : Inport  Port=14
  i14 : Inport  Port=15
  i15 : Inport  Port=16
  conv_ob0 : Subsystem
  conv_ob1 : Subsystem
  conv_ob10 : Subsystem
  conv_ob11 : Subsystem
  conv_ob12 : Subsystem
  conv_ob13 : Subsystem
  conv_ob14 : Subsystem
  conv_ob15 : Subsystem
  conv_ob2 : Subsystem
  conv_ob3 : Subsystem
  conv_ob4 : Subsystem
  conv_ob5 : Subsystem
  conv_ob6 : Subsystem
  conv_ob7 : Subsystem
  conv_ob8 : Subsystem
  conv_ob9 : Subsystem
  q0 : Outport
  q1 : Outport  Port=2
  q2 : Outport  Port=3
  q3 : Outport  Port=4
  q4 : Outport  Port=5
  q5 : Outport  Port=6
  q6 : Outport  Port=7
  q7 : Outport  Port=8
  q8 : Outport  Port=9
  q9 : Outport  Port=10
  q10 : Outport  Port=11
  q11 : Outport  Port=12
  q12 : Outport  Port=13
  q13 : Outport  Port=14
  q14 : Outport  Port=15
  q15 : Outport  Port=16
  wires:
  i0/1 -> conv_ob0/1(i)
  conv_ob0/1(q) -> q0/1
  i1/1 -> conv_ob1/1(i)
  conv_ob1/1(q) -> q1/1
  i2/1 -> conv_ob2/1(i)
  conv_ob2/1(q) -> q2/1
  i3/1 -> conv_ob3/1(i)
  conv_ob3/1(q) -> q3/1
  i4/1 -> conv_ob4/1(i)
  conv_ob4/1(q) -> q4/1
  i5/1 -> conv_ob5/1(i)
  conv_ob5/1(q) -> q5/1
  i6/1 -> conv_ob6/1(i)
  conv_ob6/1(q) -> q6/1
  i7/1 -> conv_ob7/1(i)
  conv_ob7/1(q) -> q7/1
  i8/1 -> conv_ob8/1(i)
  conv_ob8/1(q) -> q8/1
  i9/1 -> conv_ob9/1(i)
  conv_ob9/1(q) -> q9/1
  i10/1 -> conv_ob10/1(i)
  conv_ob10/1(q) -> q10/1
  i11/1 -> conv_ob11/1(i)
  conv_ob11/1(q) -> q11/1
  i12/1 -> conv_ob12/1(i)
  conv_ob12/1(q) -> q12/1
  i13/1 -> conv_ob13/1(i)
  conv_ob13/1(q) -> q13/1
  i14/1 -> conv_ob14/1(i)
  conv_ob14/1(q) -> q14/1
  i15/1 -> conv_ob15/1(i)
  conv_ob15/1(q) -> q15/1

== system cal_2adc/snapshot0 ==
  note: Generate stop
      | when in circular
      | capture mode
  note: Delay start
      | of capture
  note: ctrl:
      | bit0: Put a posedge here
      |         to enable a new capture.
      | bit1: ignore external trigger
      |         and trigger immediately.
      | bit2: ignore external write
      |         enable and capture on
      |         every FPGA clock.
      | bit3: continuously capture
      |         data until we get an
      |         external stop command.
  note: Offset in vector
      | from first element
      | captured, used
      | during circular capture
  note: Number of
      | bytes in
      | buffer and
      | done bit
  note: Number of valid
      | data samples to
      | skip after trigger
      | before starting
      | capture
  note: Value on vin
      | aligned with
      | first sample on
      | din captured
  din : Inport
  we : Inport  Port=2
  trig : Inport  Port=3
  add_del : xbsIndex_r4/Delay  rst=off  infoeditControl=Selection of Reset will increase slice count due to use of real FFs and instead of SRLs  en=off  latency=1  dbl_ovrd=off  reg_retiming=on  block_type=delay
      settings: block_version=11.4
  add_gen : Subsystem  AncestorBlock=casper_library_scopes/snapshot/add_gen  mask{counter_size=10+4+1, increment=16, nsamples=10, burst_size=0, use_dsp48=on}
      mask prompts: counter_size "Address counter size (2^?)"; increment "Address counter increment"; nsamples "Number of samples (2^?)"; burst_size "Burst size (2^?)"; use_dsp48 "dsp48 counter/s"
      mask init:
      | set_param(gcb,'LinkStatus','inactive');
      | if strcmp(use_dsp48,'on'),
      |     set_param([gcb,'/add_gen'],'implementation','DSP48');
      | else
      |     set_param([gcb,'/add_gen'],'implementation','Fabric');
      | end
  basic_ctrl : Subsystem  AncestorBlock=casper_library_scopes/snapshot/basic_ctrl  mask{dram=off, data_width=128}
      mask prompts: data_width "data width"
      mask init:
      | set_param(gcb,'LinkStatus','inactive');
      | set_param([gcb,'/dram_munge'], 'dram', dram);
  bram : Subsystem  Tag=xps:bram  AncestorBlock=xps_library/Shared BRAM  mask{arith_type=Unsigned, addr_width=10, data_width=128, reg_prim_output=on, reg_core_output=on, optimization=Minimum_Area, data_bin_pt=0, init_vals=[0:2^10-1], sample_rate=1}
      mask prompts: arith_type "Output Data Type"; addr_width "Address width"; data_width "Data Width"; reg_prim_output "Register Primitive Output"; reg_core_output "Register Core Output"; data_bin_pt "Data Binary Point"; init_vals "Initial values (simulation only)"; sample_rate "Sample rate"
      mask init:
      | shared_bram_mask;
      mask TypeOptions arith_type: Unsigned | Signed  (2's comp)
      mask TypeOptions data_width: 8 | 16 | 32 | 64 | 128
      mask TypeOptions optimization: Minimum_Area | Low_Power
  cast : xbsIndex_r4/Convert  gui_display_data_type=Fixed-point  arith_type=Unsigned  n_bits=128  bin_pt=0  float_type=Single  exp_bits=8  fraction_bits=24  quantization=Truncate  overflow=Wrap  en=off  latency=0  dbl_ovrd=off  pipeline=off  block_type=convert
      settings: block_version=11.4
  const0 : Constant  Value=0
  const1 : Constant  Value=10
  ctrl : Subsystem  Tag=xps:sw_reg  AncestorBlock=xps_library/software register  mask{numios=1, io_dir=From Processor, io_delay=0, sample_period=1, name1=reg, bitwidth1=32, arith_type1=Unsigned, bin_pt1=0}
      mask prompts: numios "Num I/Os"; io_dir "I/O direction"; io_delay "I/O delay"; sample_period "Sample period"; name1 "Name"; bitwidth1 "Bitwidth"; arith_type1 "Type"; bin_pt1 "Binary pt"
      mask init:
      | swreg_init(gcb);
      mask Callback numios: t = timer('StartDelay', 0.1); t.TimerFcn = {@swreg_cb, gcb}; start(t);
      mask TypeOptions io_dir: To Processor | From Processor
      mask Callback io_dir:
      | a = get_param(gcb, 'MaskEnables');
      | if strcmp(get_param(gcb, 'io_dir'), 'To Processor'),
      | a(4) = {'off'};
      | else
      | a(4) = {'on'};
      | end
      | set_param(gcb, 'MaskEnables', a);
      mask TypeOptions arith_type1: Unsigned | Signed  (2's comp) | Boolean
      mask Callback arith_type1:
      | a = get_param(gcb, 'MaskEnables');
      | if strcmp(get_param(gcb, 'arith_type1'), 'Boolean'),
      | set_param(gcb, 'bitwidth1', '1');
      | set_param(gcb, 'bin_pt1', '0');
      | a(6) = {'off'};
      | a(8) = {'off'};
      | else
      | a(6) = {'on'};
      | a(8) = {'on'};
      | end
      | set_param(gcb, 'MaskEnables', a);
  dat_del : xbsIndex_r4/Delay  rst=off  infoeditControl=Selection of Reset will increase slice count due to use of real FFs and instead of SRLs  en=off  latency=1  dbl_ovrd=off  reg_retiming=on  block_type=delay
      settings: block_version=11.4
  delay : Subsystem  AncestorBlock=casper_library_scopes/snapshot/delay  mask{use_dsp48=on, word_size=16}
      mask prompts: use_dsp48 "dsp48 counter/s"; word_size "word byte size?"
      mask init:
      | set_param(gcb,'LinkStatus','inactive');
      | if strcmp(use_dsp48,'on'),
      |     set_param([gcb,'/counter'],'implementation','DSP48');
      | else
      |     set_param([gcb,'/counter'],'implementation','Fabric');
      | end
  g_tr_en_cnt : Terminator
  gbram : Terminator
  gstatus : Terminator
  gval : Terminator
  never : xbsIndex_r4/Constant  const=0  gui_display_data_type=Fixed-point  arith_type=Boolean  n_bits=16  bin_pt=14  preci_type=Single  exp_width=8  frac_width=24  explicit_period=on  period=1  equ=P=C  opselect=C  inp2=PCIN>>17  opr=+  inp1=P  carry=CIN  dbl_ovrd=off  block_type=constant
  ri : xbsIndex_r4/Reinterpret  force_arith_type=on  arith_type=Unsigned  force_bin_pt=on  bin_pt=0  block_type=reinterpret
      settings: infoedit="Changes signal type without altering the binary representation.   You can changed the signal between signed and unsigned, and relocate the binary point.<br><br>Hardware notes: In hardware this block costs nothing.<br><br>Example:  Suppose the input is 6 bits wide, signed, with 2 fractional bits, and the output is forced to unsigned with 0 fractional bits.  Then an input of -2.0 (1110.00 in binary 2's complement) becomes an output of 56 (111000 in binary)."
  status : Subsystem  Tag=xps:sw_reg  AncestorBlock=xps_library/software register  mask{numios=1, io_dir=To Processor, io_delay=0, sample_period=1, name1=reg, bitwidth1=32, arith_type1=Unsigned, bin_pt1=0}
      mask prompts: numios "Num I/Os"; io_dir "I/O direction"; io_delay "I/O delay"; sample_period "Sample period"; name1 "Name"; bitwidth1 "Bitwidth"; arith_type1 "Type"; bin_pt1 "Binary pt"
      mask init:
      | swreg_init(gcb);
      mask Callback numios: t = timer('StartDelay', 0.1); t.TimerFcn = {@swreg_cb, gcb}; start(t);
      mask TypeOptions io_dir: To Processor | From Processor
      mask Callback io_dir:
      | a = get_param(gcb, 'MaskEnables');
      | if strcmp(get_param(gcb, 'io_dir'), 'To Processor'),
      | a(4) = {'off'};
      | else
      | a(4) = {'on'};
      | end
      | set_param(gcb, 'MaskEnables', a);
      mask TypeOptions arith_type1: Unsigned | Signed  (2's comp) | Boolean
      mask Callback arith_type1:
      | a = get_param(gcb, 'MaskEnables');
      | if strcmp(get_param(gcb, 'arith_type1'), 'Boolean'),
      | set_param(gcb, 'bitwidth1', '1');
      | set_param(gcb, 'bin_pt1', '0');
      | a(6) = {'off'};
      | a(8) = {'off'};
      | else
      | a(6) = {'on'};
      | a(8) = {'on'};
      | end
      | set_param(gcb, 'MaskEnables', a);
  trig_offset : Subsystem  Tag=xps:sw_reg  AncestorBlock=xps_library/software register  mask{numios=1, io_dir=From Processor, io_delay=0, sample_period=1, name1=reg, bitwidth1=32, arith_type1=Unsigned, bin_pt1=0}
      mask prompts: numios "Num I/Os"; io_dir "I/O direction"; io_delay "I/O delay"; sample_period "Sample period"; name1 "Name"; bitwidth1 "Bitwidth"; arith_type1 "Type"; bin_pt1 "Binary pt"
      mask init:
      | swreg_init(gcb);
      mask Callback numios: t = timer('StartDelay', 0.1); t.TimerFcn = {@swreg_cb, gcb}; start(t);
      mask TypeOptions io_dir: To Processor | From Processor
      mask Callback io_dir:
      | a = get_param(gcb, 'MaskEnables');
      | if strcmp(get_param(gcb, 'io_dir'), 'To Processor'),
      | a(4) = {'off'};
      | else
      | a(4) = {'on'};
      | end
      | set_param(gcb, 'MaskEnables', a);
      mask TypeOptions arith_type1: Unsigned | Signed  (2's comp) | Boolean
      mask Callback arith_type1:
      | a = get_param(gcb, 'MaskEnables');
      | if strcmp(get_param(gcb, 'arith_type1'), 'Boolean'),
      | set_param(gcb, 'bitwidth1', '1');
      | set_param(gcb, 'bin_pt1', '0');
      | a(6) = {'off'};
      | a(8) = {'off'};
      | else
      | a(6) = {'on'};
      | a(8) = {'on'};
      | end
      | set_param(gcb, 'MaskEnables', a);
  vin_const : xbsIndex_r4/Constant  const=0  gui_display_data_type=Fixed-point  arith_type=Boolean  n_bits=16  bin_pt=14  preci_type=Single  exp_width=8  frac_width=24  explicit_period=on  period=1  equ=P=C  opselect=C  inp2=PCIN>>17  opr=+  inp1=P  carry=CIN  dbl_ovrd=off  block_type=constant
      settings: block_version=11.4
  we_del : xbsIndex_r4/Delay  rst=off  infoeditControl=Selection of Reset will increase slice count due to use of real FFs and instead of SRLs  en=off  latency=1  dbl_ovrd=off  reg_retiming=on  block_type=delay
      settings: block_version=11.4
  wires:
  din/1 -> ri/1
  ri/1 -> cast/1
  cast/1 -> basic_ctrl/2(din)
  we/1 -> basic_ctrl/3(we)
  trig/1 -> basic_ctrl/4(trig)
  never/1 -> basic_ctrl/6(stopi)
  const0/1 -> ctrl/1(sim_reg)
  ctrl/1(in_reg) -> basic_ctrl/5(ctrl)
  const1/1 -> trig_offset/1(sim_reg)
  basic_ctrl/1(vout) -> delay/1(vin)
  basic_ctrl/2(dout) -> delay/2(din)
  basic_ctrl/3(we_o) -> delay/3(we)
  basic_ctrl/4(go) -> delay/4(go)
  basic_ctrl/5(stop) -> delay/5(stopi)
  basic_ctrl/6(init) -> delay/6(init)
  trig_offset/1(in_reg) -> delay/7(delay)
  delay/1(vout) -> add_gen/1(vin)
  delay/2(dout) -> add_gen/2(din)
  delay/3(we_o) -> add_gen/3(we)
  delay/4(del_go) -> add_gen/4(go)
  delay/5(stop) -> add_gen/5(cont)
  delay/6(del_init) -> add_gen/6(init)
  add_gen/5(status) -> status/1(out_reg)
  status/1(sim_out) -> gstatus/1
  vin_const/1 -> basic_ctrl/1(vin)
  add_gen/1(vout) -> gval/1
  add_gen/6(en_cnt) -> g_tr_en_cnt/1
  add_gen/2(add) -> add_del/1
  add_gen/3(dout) -> dat_del/1
  add_gen/4(we_o) -> we_del/1
  add_del/1 -> bram/1(addr)
  dat_del/1 -> bram/2(data_in)
  we_del/1 -> bram/3(we)
  bram/1(data_out) -> gbram/1
